simulink model "SAC_RL_env (no DEEN, orig)"  (R2025b)
settings: Solver=ode4  StartTime=0.0  StopTime=400  FixedStep=0.005  RelTol=1e-3  EnableMultiTasking=on
values from neighbouring files (symbols this model uses):
  dyn_obs = struct('p0', cell(1, num_dyn_obs), 'v', cell(1, num_dyn_obs), 'radius', cell(1, num_dyn_obs))    [genera_ostacoli_dinamici.m]    (also in visualizza_raggi_completo.m = scenario.dynamic_obstacles)
  initialGainsMultiplier = 15    [init_rl.m]    (also in report_agent.m; test.m; test_agent.m; train.m)
  is_validation = env.isValidation    [CustomSimulinkEnv.m]    (also in get_RL_env.m = evalin('base', 'is_validation'))
  logging = true    [train.m]    (also in train_agent.m; train_agent_precedente.m)
  max_angular_vel = double(pi)    [get_RL_env.m]
  max_deviazione_pos = 100    [get_RL_env.m]
  max_deviazione_vel = 20    [get_RL_env.m]
  max_distanza_goal = double(norm(initial_pos - scenario.map.q_goal))    [get_RL_env.m]
  max_vel = 30    [get_RL_env.m]
  num_rays = size(lidar_scan, 2)    [visualizza_raggi.m]
  tolleranza_goal = 2    [get_RL_env.m]
  Ts = 0.1    [init_rl.m]    (also in report_agent.m; test.m; test_agent.m; train.m)
undefined symbols (not defined in the file or in its folder): angControlTuning, angRateControlTuning, bounds, Controller, decyear, DiscIntNeverNeededParam, DroneMass, Dz, Gravity, initialConditions, Iz, leapyear, logPath_num, logPathValid_num, Nz, pos_goal, posControlTuning, Pz, startFlightTime, tunePositionController, UAVSampleTime, Vehicle, velControlTuning
libraries: slpidlib x14, slctrl_autotuning x8, sharedutil x4, matrix_library x4, aerolibconvert2 x3, aerolibatmos2 x2, aerolibgravity2 x2, shared6dof x2, aerolibasang x2, sensorinslib x2, deeplib x1, rllib x1
(part 1 of 5)
settings Model: DataDictionary=uavPackageDeliveryDataDict.sldd  ModifiedByFormat=The MathWorks, Inc.  SimulationMode=accelerator  PacingRate=0.110000  Creator=The MathWorks, Inc.  LastModifiedBy=The MathWorks, Inc.
settings SolverCC: AlgebraicLoopSolver=TrustRegion  AutoInsertRateTranBlk=on  MaxZcPerStep=1.0
settings DataIOCC: SaveOutput=off
settings OptimizationCC: LifeSpan=inf
settings DebuggingCC: ParameterPrecisionLossMsg=none  UnconnectedInputMsg=warning  UnconnectedOutputMsg=warning  UnconnectedLineMsg=warning  AllowSymbolicDim=off  SubsystemReferenceDiagnosticForUnitTest=warning  SFUnexpectedBacktrackingDiag=warning  SFNoUnconditionalDefaultTransitionDiag=warning  SFExecutionAtInitializationDiag=none  ArithmeticOperatorsInVariantConditions=warning
settings ModelReferenceCC: EnableRefExpFcnMdlSchedulingChecks=on  PropagateSignalLabelsOutOfModel=off
settings SFSimCC: SimUseLocalCustomCode=off  CustomCodeUndefinedFunction=UseInterfaceOnly
settings RTWCC: RTWUseLocalCustomCode=off  GPUComputeCapability=3.5  DLArmComputeVersion=19.05
settings CodeAppCC: StateflowObjectComments=on
settings GRTTargetCC: TargetLangStandard=C89/C90 (ANSI)
settings ConfigComp: CovMetricSettings=dw  CovSaveCumulativeToWorkspaceVar=on  CovSaveSingleToWorkspaceVar=on  CovExternalEMLEnable=off

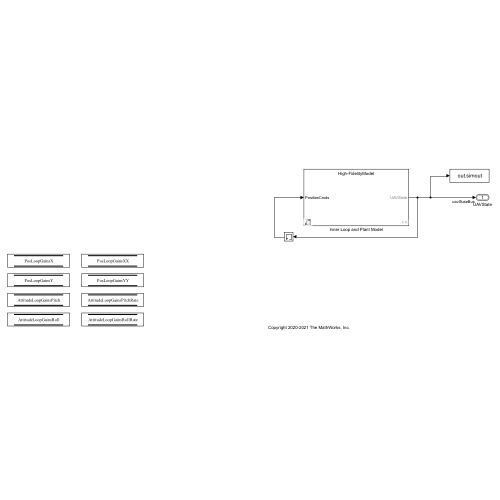
[thumbnail: Simulink's stored preview of the top-level diagram]
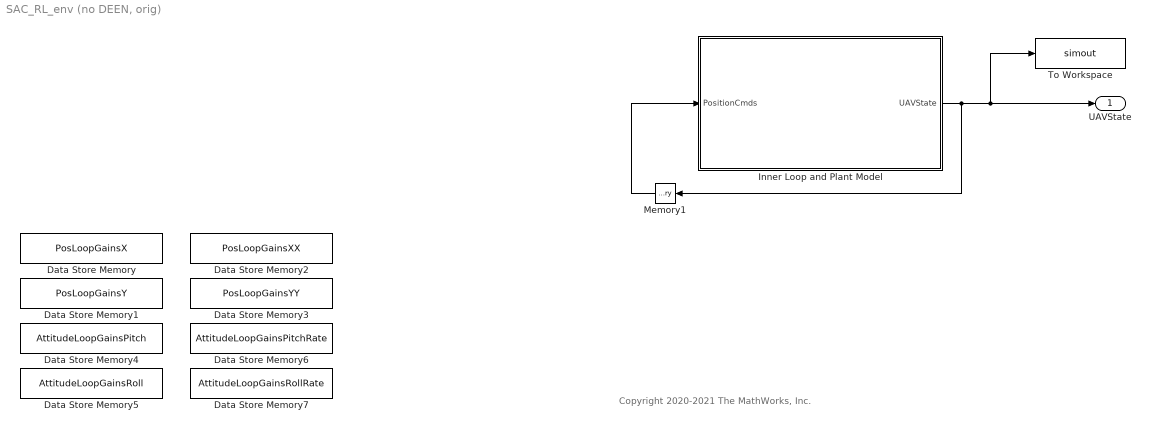
== system SAC_RL_env (no DEEN, orig) ==
  note: Copyright 2020-2021 The MathWorks, Inc.
  Data Store Memory : DataStoreMemory  DataStoreName=PosLoopGainsX  ReadBeforeWriteMsg=warning  WriteAfterWriteMsg=warning  WriteAfterReadMsg=warning  InitialValue=0.25*initialGainsMultiplier  ShowAdditionalParam=off
  Data Store Memory1 : DataStoreMemory  DataStoreName=PosLoopGainsY  ReadBeforeWriteMsg=warning  WriteAfterWriteMsg=warning  WriteAfterReadMsg=warning  InitialValue=0.25*initialGainsMultiplier  ShowAdditionalParam=off
  Data Store Memory2 : DataStoreMemory  DataStoreName=PosLoopGainsXX  ReadBeforeWriteMsg=warning  WriteAfterWriteMsg=warning  WriteAfterReadMsg=warning  InitialValue=[0.15 0.075].*initialGainsMultiplier  ShowAdditionalParam=off
  Data Store Memory3 : DataStoreMemory  DataStoreName=PosLoopGainsYY  ReadBeforeWriteMsg=warning  WriteAfterWriteMsg=warning  WriteAfterReadMsg=warning  InitialValue=[0.15 0.075].*initialGainsMultiplier  ShowAdditionalParam=off
  Data Store Memory4 : DataStoreMemory  DataStoreName=AttitudeLoopGainsPitch  ReadBeforeWriteMsg=warning  WriteAfterWriteMsg=warning  WriteAfterReadMsg=warning  InitialValue=5*initialGainsMultiplier  ShowAdditionalParam=off
  Data Store Memory5 : DataStoreMemory  DataStoreName=AttitudeLoopGainsRoll  ReadBeforeWriteMsg=warning  WriteAfterWriteMsg=warning  WriteAfterReadMsg=warning  InitialValue=5*initialGainsMultiplier  ShowAdditionalParam=off
  Data Store Memory6 : DataStoreMemory  DataStoreName=AttitudeLoopGainsPitchRate  ReadBeforeWriteMsg=warning  WriteAfterWriteMsg=warning  WriteAfterReadMsg=warning  InitialValue=[0.0025 2*0.0025 0.0025/25 70].*initialGainsMultiplier  ShowAdditionalParam=off
  Data Store Memory7 : DataStoreMemory  DataStoreName=AttitudeLoopGainsRollRate  ReadBeforeWriteMsg=warning  WriteAfterWriteMsg=warning  WriteAfterReadMsg=warning  InitialValue=[0.002 0.003 0.003/50 70].*initialGainsMultiplier  ShowAdditionalParam=off
  Inner Loop and Plant Model : Subsystem  Variant=on  PropagateVariantConditions=on
  Memory1 : Memory  InheritSampleTime=on
  To Workspace : ToWorkspace  VariableName=simout  SaveFormat=Timeseries  SampleTime=-1
  UAVState : Outport  OutDataTypeStr=Bus: uavStateBus  BusOutputAsStruct=on
  wires:
  Inner Loop and Plant Model/1(UAVState) -> Memory1/1, To Workspace/1, UAVState/1
  Memory1/1 -> Inner Loop and Plant Model/1(PositionCmds)

== system SAC_RL_env (no DEEN, orig)/Inner Loop and Plant Model ==
  PositionCmds : Inport
  High-FidelityModel : Subsystem  VariantControl=plantModelFi==1
  High-FidelityModel with Autotuning : Subsystem  VariantControl=plantModelFi==2
  Low-FidelityModel : Subsystem  VariantControl=plantModelFi ==0
  UAVState : Outport

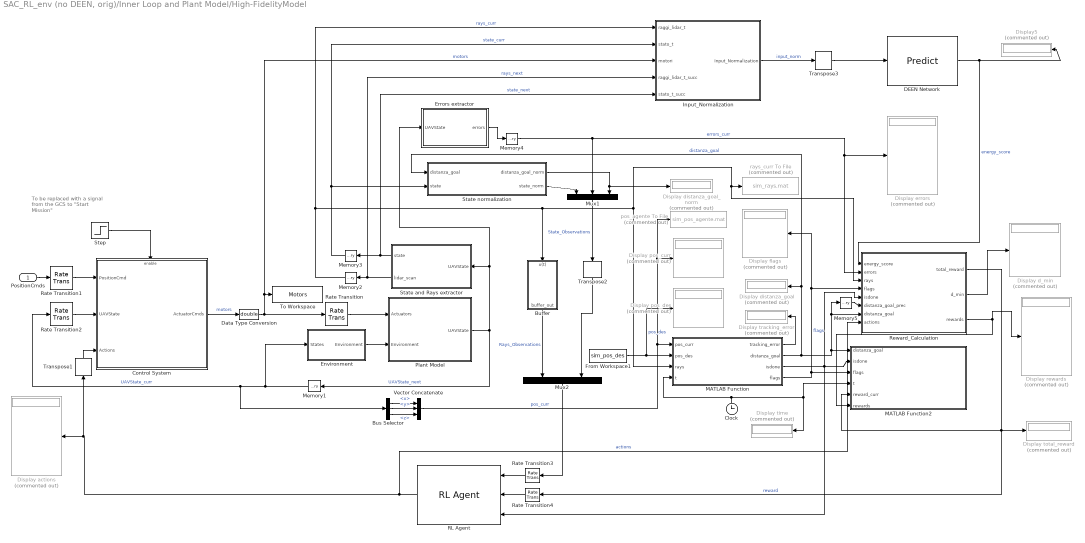
== system SAC_RL_env (no DEEN, orig)/Inner Loop and Plant Model/High-FidelityModel ==
  note: To be replaced with a signal from the GCS to "Start Mission"
  PositionCmds : Inport
  Buffer : Subsystem
  Bus Selector : BusSelector  OutputSignals=pos_vel.x,pos_vel.y,pos_vel.z
  Clock : Clock
  Control System : Subsystem  TreatAsAtomicUnit=on  SystemSampleTime=UAVSampleTime
  DEEN Network : deeplib/Predict  Network=Network from MAT-file  NetworkFunction=squeezenet  NetworkFilePath=deen_network.mat  MiniBatchSize=128  InputDataFormats={'input_transition', 'CB';}  Predictions=on  Activations={}  ForceInterpretedSim=off  EnableDLNetwork=on  LastKnownNetworkFilePath='deen_network.mat'  LastKnownNetworkTimeStamp=740118.69643518514931201934814453125
  Data Type Conversion : DataTypeConversion  OutDataTypeStr=double  SaturateOnIntegerOverflow=off  RndMeth=Floor
  Display actions : Display  Commented=on
  Display d_min : Display  Commented=on
  Display distanza_goal : Display  Commented=on
  Display distanza_goal_norm : Display  Commented=on
  Display errors : Display  Commented=on
  Display flags : Display  Commented=on
  Display pos_curr : Display  Commented=on
  Display pos_des : Display  Commented=on
  Display rewards : Display  Commented=on
  Display time : Display  Commented=on
  Display total_reward : Display  Commented=on
  Display tracking_error : Display  Commented=on
  Display5 : Display  Commented=on
  Environment : Subsystem  TreatAsAtomicUnit=on  VariantControl=VSS_ENVIRONMENT_VARIABLE
  Errors extractor : Subsystem
  From Workspace1 : FromWorkspace  VariableName=sim_pos_des
  Input_Normalization : MATLAB Function  TreatAsAtomicUnit=on
  MATLAB Function : MATLAB Function  TreatAsAtomicUnit=on
  MATLAB Function2 : MATLAB Function  TreatAsAtomicUnit=on  SystemSampleTime=Ts
  Memory{1,3..5} (4 alike) : Memory  InheritSampleTime=on  LinearizeMemory=on  LinearizeAsDelay=on
  Memory2 : Memory  InitialCondition=ones(1, num_rays)  InheritSampleTime=on  LinearizeMemory=on  LinearizeAsDelay=on
  Mux1 : Mux  Inputs=3
  Mux2 : Mux  Inputs=2
  Plant Model : Subsystem  TreatAsAtomicUnit=on
  RL Agent : rllib/RL Agent  Agent=agent  ExternalActionAsInput=off  ProvideLastAction=off  ProvideCumRwd=off  TreatAsDirectFeedthrough=on  UseStrictObservationDataTypes=off
  Rate Transition : RateTransition
  Rate Transition1 : RateTransition  OutPortSampleTime=UAVSampleTime
  Rate Transition2 : RateTransition  OutPortSampleTime=UAVSampleTime
  Rate Transition3 : RateTransition
  Rate Transition4 : RateTransition
  Reward_Calculation : MATLAB Function  TreatAsAtomicUnit=on
  State and Rays extractor : Subsystem
  State normalization : MATLAB Function  TreatAsAtomicUnit=on
  Step : Step  Time=0  SampleTime=UAVSampleTime
  To Workspace : ToWorkspace  VariableName=Motors  SaveFormat=Timeseries  SampleTime=-1
  Transpose1 : matrix_library/Transpose
  Transpose2 : matrix_library/Transpose
  Transpose3 : matrix_library/Transpose
  Vector Concatenate : Concatenate  NumInputs=3
  pos_agente To File : ToFile  Commented=on  Filename=sim_pos_agente.mat  MatrixName=sim_pos_agente  SaveFormat=Timeseries
  rays_curr To File : ToFile  Commented=on  Filename=sim_rays.mat  MatrixName=sim_rays  SaveFormat=Timeseries  SampleTime=Ts
  wires:
  PositionCmds/1 -> Rate Transition1/1
  Control System/1(ActuatorCmds) -> Data Type Conversion/1  "motors"
  Environment/1(Environment) -> Plant Model/2(Environment)
  Memory1/1 -> Bus Selector/1, Rate Transition2/1, Environment/1(States)  "UAVState_curr"
  Plant Model/1(UAVState) -> Memory1/1, State and Rays extractor/1(UAVState), Errors extractor/1(UAVState)  "UAVState_next"
  Step/1 -> Control System/Enable
  Rate Transition/1 -> Plant Model/1(Actuators)
  Rate Transition1/1 -> Control System/1(PositionCmd)
  Rate Transition2/1 -> Control System/2(UAVState)
  State and Rays extractor/2(lidar_scan) -> Input_Normalization/4(raggi_lidar_t_succ), Memory2/1  "rays_next"
  State and Rays extractor/1(state) -> Input_Normalization/5(stato_t_succ), Memory3/1  "state_next"
  Memory3/1 -> Input_Normalization/2(stato_t), State normalization/2(state)  "state_curr"
  From Workspace1/1 -> Display pos_des/1, MATLAB Function/2(pos_des)  "pos_des"
  Data Type Conversion/1 -> Input_Normalization/3(motori), To Workspace/1, Rate Transition/1  "motors"
  Bus Selector/3 -> Vector Concatenate/3  "<z>"
  Bus Selector/2 -> Vector Concatenate/2  "<y>"
  Bus Selector/1 -> Vector Concatenate/1  "<x>"
  Vector Concatenate/1 -> MATLAB Function/1(pos_curr), pos_agente To File/1, Display pos_curr/1  "pos_curr"
  RL Agent/1 -> Display actions/1, Transpose1/1, Reward_Calculation/8(actions)  "actions"
  Reward_Calculation/1(total_reward) -> Display total_reward/1, Rate Transition4/1, MATLAB Function2/5(reward_curr)  "reward"
  DEEN Network/1 -> Reward_Calculation/1(energy_score), Display5/1  "energy_score"
  Rate Transition3/1 -> RL Agent/1
  Rate Transition4/1 -> RL Agent/2
  Errors extractor/1(errors) -> Memory4/1
  Memory4/1 -> Display errors/1, Reward_Calculation/2(errors), Mux1/2  "errors_curr"
  Mux1/1 -> Transpose2/1  "State_Observations"
  Memory2/1 -> Input_Normalization/1(raggi_lidar_t), Buffer/1(x(t)), MATLAB Function/3(rays), Reward_Calculation/3(rays), rays_curr To File/1  "rays_curr"
  MATLAB Function/3(isdone) -> Reward_Calculation/5(isdone), MATLAB Function2/2(isdone), RL Agent/3
  MATLAB Function/4(flags) -> MATLAB Function2/3(flags), Display flags/1, Reward_Calculation/4(flags)  "flags"
  MATLAB Function/1(tracking_error) -> Display tracking_error/1
  Transpose1/1 -> Control System/3(Actions)
  Clock/1 -> MATLAB Function/4(t), Display time/1, MATLAB Function2/4(t)
  Buffer/1(buffer_out) -> Mux2/1  "Rays_Observations"
  Mux2/1 -> Rate Transition3/1
  State normalization/2(state_norm) -> Mux1/1
  Transpose2/1 -> Mux2/2
  Reward_Calculation/2(d_min) -> Display d_min/1
  Memory5/1 -> Reward_Calculation/6(distanza_goal_prec)
  Reward_Calculation/3(rewards) -> Display rewards/1, MATLAB Function2/6(rewards)
  Input_Normalization/1(Input_Normalization) -> Transpose3/1  "input_norm"
  MATLAB Function/2(distanza_goal) -> Display distanza_goal/1, State normalization/1(distanza_goal), Memory5/1, Reward_Calculation/7(distanza_goal), MATLAB Function2/1(distanza_goal)  "distanza_goal"
  State normalization/1(distanza_goal_norm) -> Display distanza_goal_norm/1, Mux1/3
  Transpose3/1 -> DEEN Network/1

== system SAC_RL_env (no DEEN, orig)/Inner Loop and Plant Model/High-FidelityModel with Autotuning ==
  note: To be replaced with a signal from the GCS to "Start Mission"
  PositionCmds : Inport
  Control System : Subsystem  TreatAsAtomicUnit=on  SystemSampleTime=UAVSampleTime
  Environment : Subsystem  TreatAsAtomicUnit=on  VariantControl=VSS_ENVIRONMENT_VARIABLE
  Memory1 : Memory  InheritSampleTime=on  LinearizeMemory=on  LinearizeAsDelay=on
  Plant Model : Subsystem  TreatAsAtomicUnit=on
  Rate Transition : RateTransition
  Rate Transition1 : RateTransition  OutPortSampleTime=UAVSampleTime
  Rate Transition2 : RateTransition  OutPortSampleTime=UAVSampleTime
  Step : Step  Time=startFlightTime  SampleTime=UAVSampleTime
  UAVState : Outport  OutDataTypeStr=Bus: uavStateBus
  wires:
  PositionCmds/1 -> Rate Transition1/1
  Control System/1(ActuatorCmds) -> Rate Transition/1  "motors"
  Environment/1(Environment) -> Plant Model/2(Environment)
  Memory1/1 -> Environment/1(States), Rate Transition2/1
  Plant Model/1(UAVState) -> UAVState/1, Memory1/1
  Step/1 -> Control System/Enable
  Rate Transition/1 -> Plant Model/1(Actuators)
  Rate Transition1/1 -> Control System/1(PositionCmd)
  Rate Transition2/1 -> Control System/2(UAVState)

== system SAC_RL_env (no DEEN, orig)/Inner Loop and Plant Model/Low-FidelityModel ==
  PositionCmds : Inport
  Assemble UAV State Bus : Subsystem
  Bus Creator1 : BusCreator  Inputs=1  OutDataTypeStr=Bus: uavGuidanceEnvironmentBus  NonVirtualBus=on
  Constant : Constant  Value=Gravity  OutDataTypeStr=single
      settings: AttributesFormatString=%<Value>
  Position and Acceleration Control : Subsystem
  Quadrotor Plant : uavalgslib/Guidance Model  ModelType=MultirotorGuidance  NumInstances=1  SpecifiedDataType=single  SimulateUsing=Code generation  InitialWorldPositionMultirotor=[-186; -105; 0]  InitialWorldVelocityMultirotor=[0; 0; 0]  InitialEulerZYXMultirotor=[0; 0; 0]  InitialBodyAngularRateRPYMultirotor=[0; 0; 0]  InitialThrustMultirotor=0  InitialNorthFixedWing=0  InitialEastFixedWing=0  InitialHeightFixedWing=0  InitialAirSpeedFixedWing=0  InitialHeadingAngleFixedWing=0  InitialFlightPathAngleFixedWing=0  InitialRollAngleFixedWing=0  InitialRollAngleRateFixedWing=0  PDRollMultirotor=[3402.97,116.67]  PDPitchMultirotor=[3402.97, 116.67]  PYawRateMultirotor=1950  PThrustMultirotor=39  MassMultirotor=0.1  PHeightFixedWing=3.9  PHeadingAngleFixedWing=3.9  PFlightPathAngleFixedWing=39  PDRollFixedWing=[3402.97, 116.67]  PAirSpeedFixedWing=1  FlightPathAngleLimitsFixedWing=[-pi/2, pi/2]  StateBusName='uavGuidanceStateBus'  ControlBusName='uavGuidanceControlBus'  EnvironmentBusName='uavGuidanceEnvironmentBus'  DataType=single
  Rate Transition1 : RateTransition  OutPortSampleTime=UAVSampleTime
  Rate Transition2 : RateTransition  OutPortSampleTime=UAVSampleTime
  UAVState : Outport  OutDataTypeStr=Bus: uavStateBus
  wires:
  Constant/1 -> Bus Creator1/1  "Gravity"
  Bus Creator1/1 -> Quadrotor Plant/2
  Position and Acceleration Control/1(Control Signal) -> Rate Transition2/1
  Quadrotor Plant/1 -> Rate Transition1/1
  Rate Transition2/1 -> Quadrotor Plant/1
  PositionCmds/1 -> Position and Acceleration Control/2(PositionCmd)
  Rate Transition1/1 -> Position and Acceleration Control/1(QuadRotorState), Assemble UAV State Bus/1(State)
  Assemble UAV State Bus/1(UAVState) -> UAVState/1

== system SAC_RL_env (no DEEN, orig)/Inner Loop and Plant Model/High-FidelityModel/Buffer ==
  x(t) : Inport
  Memory5 : Memory  InitialCondition=ones(1, num_rays)  InheritSampleTime=on  LinearizeMemory=on  LinearizeAsDelay=on
  Memory6 : Memory  InitialCondition=ones(1, num_rays)  InheritSampleTime=on  LinearizeMemory=on  LinearizeAsDelay=on
  Vector Concatenate1 : Concatenate  NumInputs=3
  buffer_out : Outport
  wires:
  Memory6/1 -> Vector Concatenate1/3  "x(t-2)"
  Memory5/1 -> Memory6/1, Vector Concatenate1/2  "x(t-1)"
  x(t)/1 -> Memory5/1, Vector Concatenate1/1
  Vector Concatenate1/1 -> buffer_out/1

== system SAC_RL_env (no DEEN, orig)/Inner Loop and Plant Model/High-FidelityModel/Control System ==
  note: Derived from the work by Sertac
      | Karaman and Fabian Riether
  PositionCmd : Inport
  UAVState : Inport  Port=2  BusOutputAsStruct=on
  Actions : Inport  Port=3
  Enable : EnablePort  StatesWhenEnabling=reset
  Controller : Subsystem
  ActuatorCmds : Outport  VectorParamsAs1DForOutWhenUnconnected=off
  wires:
  Controller/1(motors_refout) -> ActuatorCmds/1
  UAVState/1 -> Controller/2(UAVState)
  PositionCmd/1 -> Controller/1(PositionCmd)
  Actions/1 -> Controller/3(actions)

== system SAC_RL_env (no DEEN, orig)/Inner Loop and Plant Model/High-FidelityModel/Environment ==
  States : Inport
  Bus Creator : BusCreator  Inputs=3  OutDataTypeStr=Bus: EnvironmentBus  NonVirtualBus=on
  Bus Creator1 : BusCreator  Inputs=4  OutDataTypeStr=Bus: AtmosphereBus  NonVirtualBus=on
  Bus Selector : BusSelector  OutputSignals=gps.lat,gps.lon,gps.alt
  COESA Atmosphere Model : aerolibatmos2/COESA Atmosphere Model  units=Metric (MKS)  spec=1976 COESA-extended U.S. Standard Atmosphere  model=Profile  profile_var=High temperature  profile_percent=1%  profile_alt=5 km (16404 ft)  envelope_var=High temperature  envelope_percent=1%  action=None
  Clock : Clock
  Gain : Gain  Gain=1/1e7  OutDataTypeStr=double
  Gain1 : Gain  Gain=1/1e7  OutDataTypeStr=double
  Gain2 : Gain  Gain=1/-1e3  OutDataTypeStr=double
  Initial date : Constant  Value=decyear(initialConditions.date)
  Mux : Mux  Inputs=3
  Sum : Sum  Inputs=|++
  "WGS84 Gravity Model  " : GravityWGS84  action=None
  World Magnetic Model 2015 : aerolibgravity2/World Magnetic Model  model=WMM2015 V2 (2015-2020)  customFile='WMM2020.COF'  units=Metric (MKS)  time_in=on  month=January  day=1  year=2015  action=Error  h_out=off  dec_out=off  inc_out=off  ti_out=off
  kclock : Gain  Gain=1/(60*60*24*(365 + leapyear(initialConditions.date(1))))
  Environment : Outport  VectorParamsAs1DForOutWhenUnconnected=off
  wires:
  States/1 -> Bus Selector/1  "StatesLog"
  Bus Creator/1 -> Environment/1
  COESA Atmosphere Model/1 -> Bus Creator1/1  "air_temp"
  COESA Atmosphere Model/2 -> Bus Creator1/2  "speed_sound"
  COESA Atmosphere Model/3 -> Bus Creator1/3  "pressure"
  COESA Atmosphere Model/4 -> Bus Creator1/4  "air_density"
  Bus Creator1/1 -> Bus Creator/2  "AtmosphereBus"
  World Magnetic Model 2015/1 -> Bus Creator/3  "MagneticField_ned"
  "WGS84 Gravity Model  "/1 -> Bus Creator/1  "Gravity_ned"
  Clock/1 -> kclock/1
  Initial date/1 -> Sum/1
  Sum/1 -> World Magnetic Model 2015/4
  kclock/1 -> Sum/2
  Mux/1 -> "WGS84 Gravity Model  "/1
  Gain/1 -> World Magnetic Model 2015/2, Mux/1
  Bus Selector/1 -> Gain/1  "<lat>"
  Bus Selector/2 -> Gain1/1  "<lon>"
  Gain1/1 -> World Magnetic Model 2015/3, Mux/2
  Bus Selector/3 -> Gain2/1  "<alt>"
  Gain2/1 -> COESA Atmosphere Model/1, World Magnetic Model 2015/1, Mux/3

== system SAC_RL_env (no DEEN, orig)/Inner Loop and Plant Model/High-FidelityModel/Errors extractor ==
  UAVState : Inport
  Bus Selector3 : BusSelector  OutputSignals=pos_vel.vx,pos_vel.vy,pos_vel.vz
  Bus Selector4 : BusSelector  Commented=on  OutputSignals=attitude.yaw
  Bus Selector5 : BusSelector  OutputSignals=pos_vel.x,pos_vel.y,pos_vel.z
  Errors normalization : MATLAB Function  TreatAsAtomicUnit=on
  From Workspace3 : FromWorkspace  VariableName=sim_pos_des
  From Workspace4 : FromWorkspace  VariableName=sim_vel_des
  From Workspace5 : FromWorkspace  Commented=on  VariableName=sim_yaw_des
  Subtract : Sum  Inputs=+-
  Subtract1 : Sum  Inputs=+-
  Subtract2 : Sum  Commented=on  Inputs=+-
  Vector Concatenate5 : Concatenate
  Vector Concatenate4 : Concatenate  NumInputs=3
  Vector Concatenate6 : Concatenate  NumInputs=3
  errors : Outport  OutDataTypeStr=double
  wires:
  From Workspace4/1 -> Subtract1/1  "vel_des"
  Vector Concatenate6/1 -> Subtract/2
  Bus Selector3/1 -> Vector Concatenate4/1  "<vx>"
  Bus Selector3/2 -> Vector Concatenate4/2  "<vy>"
  Vector Concatenate4/1 -> Subtract1/2
  From Workspace3/1 -> Subtract/1
  Bus Selector5/1 -> Vector Concatenate6/1  "<x>"
  From Workspace5/1 -> Subtract2/1  "yaw_des"
  Bus Selector4/1 -> Subtract2/2  "<yaw>"
  Bus Selector5/3 -> Vector Concatenate6/3  "<z>"
  UAVState/1 -> Bus Selector5/1, Bus Selector3/1, Bus Selector4/1
  Subtract1/1 -> Vector Concatenate5/2  "errore_vel"
  Subtract/1 -> Vector Concatenate5/1  "errore_pos"
  Bus Selector5/2 -> Vector Concatenate6/2  "<y>"
  Vector Concatenate5/1 -> Errors normalization/1(errors)
  Bus Selector3/3 -> Vector Concatenate4/3  "<vz>"
  Subtract2/1 -> ?  "errore_yaw"
  Errors normalization/1(errors_normalized) -> errors/1

== system SAC_RL_env (no DEEN, orig)/Inner Loop and Plant Model/High-FidelityModel/Plant Model ==
  Actuators : Inport
  Environment : Inport  Port=2
  6DOF (Quaternion) : shared6dof/6DOF (Euler Angles)  units=Metric (MKS)  mtype=Fixed  rep=Euler Angles  xme_0=init_pos  Vm_0=[0 0 0]  eul_0=[0,0,0]  pm_0=[0,0,0]  mass_0=Vehicle.Airframe.mass  mass_e=0.5  mass_f=2.0  inertia=Vehicle.Airframe.inertia  inertia_e=eye(3)  inertia_f=2*eye(3)  k_quat=Vehicle.SixDOF.quatGain  vre_flag=on  abi_flag=on  aMode=aMode  xme_statename=''  Vm_statename=''  eul_statename=''  quat_statename=''  pm_statename=''  mass_statename=''
  AC model : Subsystem
  Bus setup : Subsystem
  Direction Cosine Matrix to Quaternions : Dcm2Quat
  Terminator1 : Terminator
  Terminator2 : Terminator
  Terminator3 : Terminator
  To Workspace : ToWorkspace  VariableName=quat_sim  SaveFormat=Timeseries  SampleTime=-1
  UAVState : Outport  VectorParamsAs1DForOutWhenUnconnected=off
  wires:
  Actuators/1 -> AC model/1(Actuators)
  Environment/1 -> AC model/2(Environment)
  AC model/1(F_cg) -> 6DOF (Quaternion)/1
  AC model/2(M_cg) -> 6DOF (Quaternion)/2
  6DOF (Quaternion)/1 -> Bus setup/1(V_ned)
  6DOF (Quaternion)/2 -> Bus setup/2(X_ned)
  6DOF (Quaternion)/3 -> Bus setup/3(Euler)
  6DOF (Quaternion)/6 -> Bus setup/5(Omega_b), AC model/5(w_b)
  6DOF (Quaternion)/5 -> AC model/4(V_b)
  6DOF (Quaternion)/4 -> Bus setup/4(DCM), Direction Cosine Matrix to Quaternions/1, AC model/3(DCM_be)
  Bus setup/1(UAVState) -> UAVState/1
  6DOF (Quaternion)/9 -> Terminator1/1
  6DOF (Quaternion)/7 -> Terminator2/1
  6DOF (Quaternion)/8 -> Terminator3/1
  Direction Cosine Matrix to Quaternions/1 -> To Workspace/1

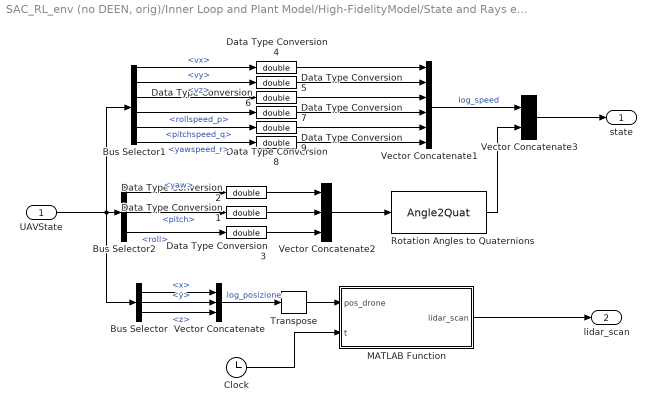
== system SAC_RL_env (no DEEN, orig)/Inner Loop and Plant Model/High-FidelityModel/State and Rays extractor ==
  UAVState : Inport
  Bus Selector : BusSelector  OutputSignals=pos_vel.x,pos_vel.y,pos_vel.z
  Bus Selector1 : BusSelector  OutputSignals=pos_vel.vx,pos_vel.vy,pos_vel.vz,attitude.rollspeed_p,attitude.pitchspeed_q,attitude.yawspeed_r
  Bus Selector2 : BusSelector  OutputSignals=attitude.yaw,attitude.pitch,attitude.roll
  Clock : Clock
  Data Type Conversion{1..9} (9 alike) : DataTypeConversion  OutDataTypeStr=double  SaturateOnIntegerOverflow=off  RndMeth=Floor
  MATLAB Function : MATLAB Function  TreatAsAtomicUnit=on
  Rotation Angles to Quaternions : Angle2Quat
      settings: AttributesFormatString=Rotation Order: %<rotationOrder>
  Transpose : matrix_library/Transpose
  Vector Concatenate : Concatenate  NumInputs=3
  Vector Concatenate1 : Concatenate  NumInputs=6
  Vector Concatenate2 : Concatenate  NumInputs=3
  Vector Concatenate3 : Concatenate
  state : Outport  OutDataTypeStr=double
  lidar_scan : Outport  Port=2  OutDataTypeStr=double
  wires:
  Vector Concatenate1/1 -> Vector Concatenate3/1  "log_speed"
  Bus Selector1/1 -> Data Type Conversion4/1  "<vx>"
  Rotation Angles to Quaternions/1 -> Vector Concatenate3/2
  Bus Selector1/4 -> Data Type Conversion7/1  "<rollspeed_p>"
  UAVState/1 -> Bus Selector2/1, Bus Selector/1, Bus Selector1/1
  Bus Selector1/2 -> Data Type Conversion5/1  "<vy>"
  Bus Selector1/5 -> Data Type Conversion8/1  "<pitchspeed_q>"
  Vector Concatenate/1 -> Transpose/1  "log_posizione"
  Bus Selector/1 -> Vector Concatenate/1  "<x>"
  Bus Selector1/3 -> Data Type Conversion6/1  "<vz>"
  Bus Selector1/6 -> Data Type Conversion9/1  "<yawspeed_r>"
  Vector Concatenate2/1 -> Rotation Angles to Quaternions/1
  Bus Selector/3 -> Vector Concatenate/3  "<z>"
  Bus Selector/2 -> Vector Concatenate/2  "<y>"
  Vector Concatenate3/1 -> state/1
  Bus Selector2/2 -> Data Type Conversion1/1  "<pitch>"
  Data Type Conversion1/1 -> Vector Concatenate2/2
  Bus Selector2/1 -> Data Type Conversion2/1  "<yaw>"
  Data Type Conversion2/1 -> Vector Concatenate2/1
  Data Type Conversion3/1 -> Vector Concatenate2/3
  Bus Selector2/3 -> Data Type Conversion3/1  "<roll>"
  Data Type Conversion4/1 -> Vector Concatenate1/1
  Data Type Conversion5/1 -> Vector Concatenate1/2
  Data Type Conversion6/1 -> Vector Concatenate1/3
  Data Type Conversion7/1 -> Vector Concatenate1/4
  Data Type Conversion8/1 -> Vector Concatenate1/5
  Data Type Conversion9/1 -> Vector Concatenate1/6
  Transpose/1 -> MATLAB Function/1(pos_drone)
  Clock/1 -> MATLAB Function/2(t)
  MATLAB Function/1(lidar_scan) -> lidar_scan/1

== system SAC_RL_env (no DEEN, orig)/Inner Loop and Plant Model/High-FidelityModel with Autotuning/Control System ==
  note: Derived from the work by Sertac
      | Karaman and Fabian Riether
  PositionCmd : Inport
  UAVState : Inport  Port=2  BusOutputAsStruct=on
  Enable : EnablePort  StatesWhenEnabling=reset
  Controller : Subsystem
  ActuatorCmds : Outport  VectorParamsAs1DForOutWhenUnconnected=off
  wires:
  Controller/1(motors_refout) -> ActuatorCmds/1
  UAVState/1 -> Controller/2(UAVState)
  PositionCmd/1 -> Controller/1(PositionCmd)

== system SAC_RL_env (no DEEN, orig)/Inner Loop and Plant Model/High-FidelityModel with Autotuning/Environment ==
  States : Inport
  Bus Creator : BusCreator  Inputs=3  OutDataTypeStr=Bus: EnvironmentBus  NonVirtualBus=on
  Bus Creator1 : BusCreator  Inputs=4  OutDataTypeStr=Bus: AtmosphereBus  NonVirtualBus=on
  Bus Selector : BusSelector  OutputSignals=gps.lat,gps.lon,gps.alt
  COESA Atmosphere Model : aerolibatmos2/COESA Atmosphere Model  units=Metric (MKS)  spec=1976 COESA-extended U.S. Standard Atmosphere  model=Profile  profile_var=High temperature  profile_percent=1%  profile_alt=5 km (16404 ft)  envelope_var=High temperature  envelope_percent=1%  action=None
  Clock : Clock
  Gain : Gain  Gain=1/1e7  OutDataTypeStr=double
  Gain1 : Gain  Gain=1/1e7  OutDataTypeStr=double
  Gain2 : Gain  Gain=1/-1e3  OutDataTypeStr=double
  Initial date : Constant  Value=decyear(initialConditions.date)
  Mux : Mux  Inputs=3
  Sum : Sum  Inputs=|++
  "WGS84 Gravity Model  " : GravityWGS84  action=None
  World Magnetic Model 2015 : aerolibgravity2/World Magnetic Model  model=WMM2015 V2 (2015-2020)  customFile='WMM2020.COF'  units=Metric (MKS)  time_in=on  month=January  day=1  year=2015  action=Error  h_out=off  dec_out=off  inc_out=off  ti_out=off
  kclock : Gain  Gain=1/(60*60*24*(365 + leapyear(initialConditions.date(1))))
  Environment : Outport  VectorParamsAs1DForOutWhenUnconnected=off
  wires:
  States/1 -> Bus Selector/1  "StatesLog"
  Bus Creator/1 -> Environment/1
  COESA Atmosphere Model/1 -> Bus Creator1/1  "air_temp"
  COESA Atmosphere Model/2 -> Bus Creator1/2  "speed_sound"
  COESA Atmosphere Model/3 -> Bus Creator1/3  "pressure"
  COESA Atmosphere Model/4 -> Bus Creator1/4  "air_density"
  Bus Creator1/1 -> Bus Creator/2  "AtmosphereBus"
  World Magnetic Model 2015/1 -> Bus Creator/3  "MagneticField_ned"
  "WGS84 Gravity Model  "/1 -> Bus Creator/1  "Gravity_ned"
  Clock/1 -> kclock/1
  Initial date/1 -> Sum/1
  Sum/1 -> World Magnetic Model 2015/4
  kclock/1 -> Sum/2
  Mux/1 -> "WGS84 Gravity Model  "/1
  Gain/1 -> World Magnetic Model 2015/2, Mux/1
  Bus Selector/1 -> Gain/1  "<lat>"
  Bus Selector/2 -> Gain1/1  "<lon>"
  Gain1/1 -> World Magnetic Model 2015/3, Mux/2
  Bus Selector/3 -> Gain2/1  "<alt>"
  Gain2/1 -> COESA Atmosphere Model/1, World Magnetic Model 2015/1, Mux/3

== system SAC_RL_env (no DEEN, orig)/Inner Loop and Plant Model/High-FidelityModel with Autotuning/Plant Model ==
  Actuators : Inport
  Environment : Inport  Port=2
  6DOF (Quaternion) : shared6dof/6DOF (Euler Angles)  units=Metric (MKS)  mtype=Fixed  rep=Euler Angles  xme_0=initialConditions.posNED + [0 0 -1]  Vm_0=[0 0 0]  eul_0=[0,0,0]  pm_0=[0,0,0]  mass_0=Vehicle.Airframe.mass  mass_e=0.5  mass_f=2.0  inertia=Vehicle.Airframe.inertia  inertia_e=eye(3)  inertia_f=2*eye(3)  k_quat=Vehicle.SixDOF.quatGain  vre_flag=on  abi_flag=on  aMode=aMode  xme_statename=''  Vm_statename=''  eul_statename=''  quat_statename=''  pm_statename=''  mass_statename=''
  AC model : Subsystem
  Bus setup : Subsystem
  Terminator1 : Terminator
  Terminator2 : Terminator
  Terminator3 : Terminator
  UAVState : Outport  VectorParamsAs1DForOutWhenUnconnected=off
  wires:
  Actuators/1 -> AC model/1(Actuators)
  Environment/1 -> AC model/2(Environment)
  AC model/1(F_cg) -> 6DOF (Quaternion)/1
  AC model/2(M_cg) -> 6DOF (Quaternion)/2
  6DOF (Quaternion)/1 -> Bus setup/1(V_ned)
  6DOF (Quaternion)/2 -> Bus setup/2(X_ned)
  6DOF (Quaternion)/3 -> Bus setup/3(Euler)
  6DOF (Quaternion)/6 -> Bus setup/5(Omega_b), AC model/5(w_b)
  6DOF (Quaternion)/5 -> AC model/4(V_b)
  6DOF (Quaternion)/4 -> Bus setup/4(DCM), AC model/3(DCM_be)
  Bus setup/1(UAVState) -> UAVState/1
  6DOF (Quaternion)/9 -> Terminator1/1
  6DOF (Quaternion)/7 -> Terminator2/1
  6DOF (Quaternion)/8 -> Terminator3/1

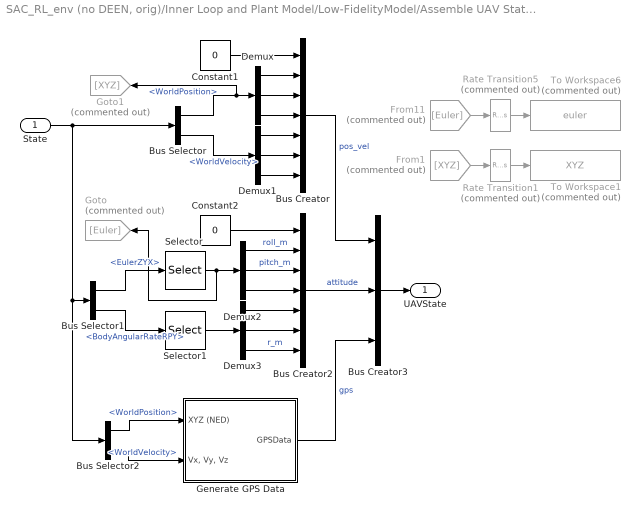
== system SAC_RL_env (no DEEN, orig)/Inner Loop and Plant Model/Low-FidelityModel/Assemble UAV State Bus ==
  State : Inport
  Bus Creator : BusCreator  Inputs=7  OutDataTypeStr=Bus: local_position_ned
      settings: InheritFromInputs=off
  Bus Creator2 : BusCreator  Inputs=7  OutDataTypeStr=Bus: attitudeBus
      settings: InheritFromInputs=off
  Bus Creator3 : BusCreator  Inputs=3  OutDataTypeStr=Bus: uavStateBus
      settings: InheritFromInputs=off
  Bus Selector : BusSelector  OutputSignals=WorldPosition,WorldVelocity
  Bus Selector1 : BusSelector  OutputSignals=EulerZYX,BodyAngularRateRPY
  Bus Selector2 : BusSelector  OutputSignals=WorldPosition,WorldVelocity
  Constant1 : Constant  Value=0  OutDataTypeStr=uint32
  Constant2 : Constant  Value=0  OutDataTypeStr=uint32
  Demux{,1..3} (4 alike) : Demux  Outputs=3
  From1 : From  Commented=on  GotoTag=XYZ
  From11 : From  Commented=on  GotoTag=Euler
  Generate GPS Data : Subsystem
  Goto : Goto  Commented=on  GotoTag=Euler
  Goto1 : Goto  Commented=on  GotoTag=XYZ
  Rate Transition1 : RateTransition  Commented=on  OutPortSampleTime=UAVSampleTime
  Rate Transition5 : RateTransition  Commented=on  OutPortSampleTime=UAVSampleTime
  Selector : Selector  InputPortWidth=3  IndexOptions=Index vector (dialog)  Indices=[3 2 1]  OutputSizes=1
  Selector1 : Selector  InputPortWidth=3  IndexOptions=Index vector (dialog)  Indices=[3 2 1]  OutputSizes=1
  To Workspace1 : ToWorkspace  Commented=on  VariableName=XYZ  SaveFormat=Timeseries  SampleTime=-1
  To Workspace6 : ToWorkspace  Commented=on  VariableName=euler  SaveFormat=Timeseries  SampleTime=-1
  UAVState : Outport  OutDataTypeStr=Bus: uavStateBus
  wires:
  Bus Creator2/1 -> Bus Creator3/2  "attitude"
  Bus Creator3/1 -> UAVState/1
  Demux3/1 -> Bus Creator2/5
  Demux1/2 -> Bus Creator/6
  Bus Creator/1 -> Bus Creator3/1  "pos_vel"
  Demux1/3 -> Bus Creator/7
  Bus Selector2/2 -> Generate GPS Data/2("Vx, Vy, Vz")  "<WorldVelocity>"
  Demux/1 -> Bus Creator/2
  State/1 -> Bus Selector/1, Bus Selector2/1, Bus Selector1/1
  Constant2/1 -> Bus Creator2/1
  Bus Selector/1 -> Goto1/1, Demux/1  "<WorldPosition>"
  Selector1/1 -> Demux3/1
  Demux1/1 -> Bus Creator/5
  Bus Selector1/1 -> Selector/1  "<EulerZYX>"
  Demux/2 -> Bus Creator/3
  Demux2/1 -> Bus Creator2/2  "roll_m"
  Demux2/3 -> Bus Creator2/4
  Demux3/2 -> Bus Creator2/6
  Demux2/2 -> Bus Creator2/3  "pitch_m"
  Bus Selector1/2 -> Selector1/1  "<BodyAngularRateRPY>"
  Demux3/3 -> Bus Creator2/7  "r_m"
  Demux/3 -> Bus Creator/4
  Bus Selector/2 -> Demux1/1  "<WorldVelocity>"
  Constant1/1 -> Bus Creator/1
  Bus Selector2/1 -> Generate GPS Data/1(XYZ (NED))  "<WorldPosition>"
  Generate GPS Data/1(GPSData) -> Bus Creator3/3  "gps"
  Rate Transition5/1 -> To Workspace6/1
  From11/1 -> Rate Transition5/1
  Selector/1 -> Goto/1, Demux2/1
  From1/1 -> Rate Transition1/1
  Rate Transition1/1 -> To Workspace1/1

== system SAC_RL_env (no DEEN, orig)/Inner Loop and Plant Model/Low-FidelityModel/Position and Acceleration Control ==
  note: To be replaced with a signal from the GCS to "Start Mission"
  QuadRotorState : Inport
  PositionCmd : Inport  Port=2
  Attitude Control : Subsystem
  Position Control : Subsystem
  Step : Step  Time=startFlightTime  SampleTime=UAVSampleTime
  Velocity Control : Subsystem
  Control Signal : Outport
  wires:
  PositionCmd/1 -> Position Control/1(PositionCmd), Attitude Control/3(PositionCmd)
  Velocity Control/1(Accel Cmd) -> Attitude Control/1(Accel Cmd)
  Attitude Control/1(Control Signal) -> Control Signal/1
  QuadRotorState/1 -> Velocity Control/2(QuadRotorState), Attitude Control/2(QuadRotorState), Position Control/2(QuadRotorState)
  Position Control/1(Velocity Cmd) -> Velocity Control/1(Velocity Cmd)
  Step/1 -> Velocity Control/Enable, Position Control/Enable

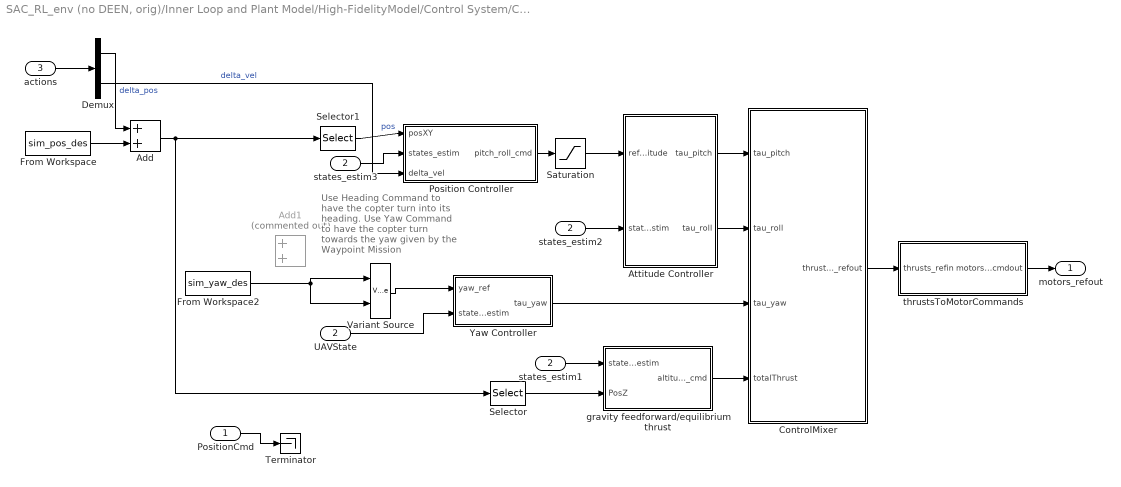
== system SAC_RL_env (no DEEN, orig)/Inner Loop and Plant Model/High-FidelityModel/Control System/Controller ==
  note: Use Heading Command to have
      | the copter turn into its heading.
      | Use Yaw Command to have the
      | copter turn towards the yaw given
      | by the Waypoint Mission
  PositionCmd : Inport
  UAVState : Inport  Port=2
  actions : Inport  Port=3
  Add : Sum
  Add1 : Sum  Commented=on
  Attitude Controller : Subsystem
  ControlMixer : Subsystem
  Demux : Demux  Outputs=[3, 3]
  From Workspace : FromWorkspace  VariableName=sim_pos_des
  From Workspace2 : FromWorkspace  VariableName=sim_yaw_des
  Position Controller : Subsystem
  Saturation : Saturate
  Selector : Selector  InputPortWidth=3  IndexOptions=Index vector (dialog)  Indices=3  OutputSizes=1
  Selector1 : Selector  InputPortWidth=3  IndexOptions=Index vector (dialog)  Indices=[1 2]  OutputSizes=1
  Terminator : Terminator
  Variant Source : VariantSource  VariantControls={useHeading ==1, useHeading~=1}
  Yaw Controller : Subsystem
  gravity feedforward/equilibrium thrust : Subsystem
  states_estim1 : InportShadow  Port=2
  states_estim2 : InportShadow  Port=2
  states_estim3 : InportShadow  Port=2
  thrustsToMotorCommands : Subsystem
  motors_refout : Outport  VectorParamsAs1DForOutWhenUnconnected=off
  wires:
  Yaw Controller/1(tau_yaw) -> ControlMixer/3(tau_yaw)
  thrustsToMotorCommands/1(motors_cmdout) -> motors_refout/1
  states_estim3/1 -> Position Controller/2(states_estim)
  ControlMixer/1(thrusts_refout) -> thrustsToMotorCommands/1(thrusts_refin)
  gravity feedforward/equilibrium thrust/1(altitude_cmd) -> ControlMixer/4(totalThrust)
  Selector1/1 -> Position Controller/1(posXY)  "pos"
  states_estim1/1 -> gravity feedforward/equilibrium thrust/1(states_estim)
  UAVState/1 -> Yaw Controller/2(states_estim)
  states_estim2/1 -> Attitude Controller/2(states_estim)
  Selector/1 -> gravity feedforward/equilibrium thrust/2(PosZ)
  Attitude Controller/1(tau_pitch) -> ControlMixer/1(tau_pitch)
  Attitude Controller/2(tau_roll) -> ControlMixer/2(tau_roll)
  Position Controller/1(pitch_roll_cmd) -> Saturation/1
  Variant Source/1 -> Yaw Controller/1(yaw_ref)
  PositionCmd/1 -> Terminator/1
  Saturation/1 -> Attitude Controller/1(refAttitude)
  From Workspace/1 -> Add/2
  Add/1 -> Selector/1, Selector1/1
  Demux/2 -> Position Controller/3(delta_vel)  "delta_vel"
  Demux/1 -> Add/1  "delta_pos"
  ? -> Add1/1  "delta_yaw"
  From Workspace2/1 -> Variant Source/1, Variant Source/2
  actions/1 -> Demux/1

== system SAC_RL_env (no DEEN, orig)/Inner Loop and Plant Model/High-FidelityModel/Plant Model/AC model ==
  Actuators : Inport
  Environment : Inport  Port=2
  DCM_be : Inport  Port=3
  V_b : Inport  Port=4  Unit=m/s
  w_b : Inport  Port=5  Unit=rad/s
  Applied Force Calculation : Subsystem
  Bus Selector : BusSelector  OutputSignals=Gravity_ned,AtmosphereBus.air_density
  Drag Calculation : Subsystem
  Gravity Force Calculation : Subsystem
  Motor Forces and Torques : Subsystem
  F_cg : Outport  Unit=N  VectorParamsAs1DForOutWhenUnconnected=off
  M_cg : Outport  Port=2  Unit=N*m  VectorParamsAs1DForOutWhenUnconnected=off
  wires:
  Applied Force Calculation/1(External Forces) -> F_cg/1
  Motor Forces and Torques/2(Motor Torques) -> M_cg/1
  Motor Forces and Torques/1(Motor Forces) -> Applied Force Calculation/3(Motor Forces)
  Bus Selector/1 -> Gravity Force Calculation/2(gravity)  "<Gravity_ned>"
  Gravity Force Calculation/1(gravity force) -> Applied Force Calculation/1(gravity force)
  Environment/1 -> Bus Selector/1
  Bus Selector/2 -> Motor Forces and Torques/2(Density), Drag Calculation/1(Density)  "<air_density>"
  DCM_be/1 -> Gravity Force Calculation/1(DCMbe)
  V_b/1 -> Motor Forces and Torques/1(Vb), Drag Calculation/2(Vb)
  Drag Calculation/1(Drag) -> Applied Force Calculation/2(Aerodynamic Forces)
  Actuators/1 -> Motor Forces and Torques/4(Motor Commands)
  w_b/1 -> Motor Forces and Torques/3(pqr)

== system SAC_RL_env (no DEEN, orig)/Inner Loop and Plant Model/High-FidelityModel/Plant Model/Bus setup ==
  V_ned : Inport  Unit=m/second  PortDimensions=3
  X_ned : Inport  Port=2  Unit=m  PortDimensions=3
  Euler : Inport  Port=3  Unit=rad  PortDimensions=3
  DCM : Inport  Port=4
  Omega_b : Inport  Port=5  Unit=rad/s  PortDimensions=3
  Bus Creator : BusCreator  Inputs=7  OutDataTypeStr=Bus: local_position_ned
      settings: InheritFromInputs=off
  Bus Creator2 : BusCreator  Inputs=7  OutDataTypeStr=Bus: attitudeBus
      settings: InheritFromInputs=off
  Bus Creator3 : BusCreator  Inputs=3  OutDataTypeStr=Bus: uavStateBus
      settings: InheritFromInputs=off
  Constant1 : Constant  Value=0  OutDataTypeStr=uint32
  Constant2 : Constant  Value=0  OutDataTypeStr=uint32
  Data Type Conversion{,1..4} (5 alike) : DataTypeConversion  OutDataTypeStr=single  SaturateOnIntegerOverflow=off  RndMeth=Floor
  Demux{,1..3} (4 alike) : Demux  Outputs=3
  Generate GPS Data : Subsystem
  UAVState : Outport  OutDataTypeStr=Bus: uavStateBus
  wires:
  Demux1/3 -> Bus Creator/7
  Bus Creator3/1 -> UAVState/1
  Demux/2 -> Bus Creator/3
  Demux3/2 -> Bus Creator2/6
  Bus Creator2/1 -> Bus Creator3/2  "attitude"
  Demux1/2 -> Bus Creator/6
  Demux3/1 -> Bus Creator2/5
  Demux/1 -> Bus Creator/2
  Euler/1 -> Data Type Conversion1/1
  Demux2/3 -> Bus Creator2/4
  Demux2/1 -> Bus Creator2/2  "roll_m"
  Bus Creator/1 -> Bus Creator3/1  "pos_vel"
  Constant2/1 -> Bus Creator2/1
  Demux2/2 -> Bus Creator2/3  "pitch_m"
  Demux3/3 -> Bus Creator2/7  "r_m"
  Demux1/1 -> Bus Creator/5
  V_ned/1 -> Data Type Conversion3/1
  Omega_b/1 -> Data Type Conversion2/1
  Demux/3 -> Bus Creator/4
  Constant1/1 -> Bus Creator/1
  Generate GPS Data/1(GPSData) -> Bus Creator3/3  "gps"
  X_ned/1 -> Data Type Conversion/1
  Data Type Conversion/1 -> Generate GPS Data/1(XYZ (NEU)), Demux/1
  Data Type Conversion2/1 -> Demux3/1
  Data Type Conversion1/1 -> Demux2/1
  Data Type Conversion3/1 -> Demux1/1, Generate GPS Data/2("Vx, Vy, Vz")
  DCM/1 -> Data Type Conversion4/1
  Data Type Conversion4/1 -> Generate GPS Data/3(DCM)

== system SAC_RL_env (no DEEN, orig)/Inner Loop and Plant Model/High-FidelityModel with Autotuning/Control System/Controller ==
  note: Use Heading Command to have
      | the copter turn into its heading.
      | Use Yaw Command to have the
      | copter turn towards the yaw given
      | by the Waypoint Mission
  In Bus Element2 : Inport  PortName=PositionCmd  Element=LAP
  In Bus Element : Inport  PortName=PositionCmd  Element=LAP
  In Bus Element3 : Inport  PortName=PositionCmd  Element=YawCmd
  In Bus Element1 : Inport  PortName=PositionCmd  Element=HeadingCmd
  UAVState : Inport  Port=2
  Attitude Controller : Subsystem
  ControlMixer : Subsystem
  Position Controller : Subsystem
  Selector : Selector  InputPortWidth=3  IndexOptions=Index vector (dialog)  Indices=3  OutputSizes=1
  Selector1 : Selector  InputPortWidth=3  IndexOptions=Index vector (dialog)  Indices=[1 2]  OutputSizes=1
  Variant Source : VariantSource  VariantControls={useHeading ==1, useHeading~=1}
  Yaw Controller : Subsystem
  gravity feedforward/equilibrium thrust : Subsystem
  states_estim1 : InportShadow  Port=2
  states_estim2 : InportShadow  Port=2
  states_estim3 : InportShadow  Port=2
  thrustsToMotorCommands : Subsystem
  motors_refout : Outport  VectorParamsAs1DForOutWhenUnconnected=off
  wires:
  Yaw Controller/1(tau_yaw) -> ControlMixer/3(tau_yaw)
  thrustsToMotorCommands/1(motors_cmdout) -> motors_refout/1
  states_estim3/1 -> Position Controller/2(states_estim)
  ControlMixer/1(thrusts_refout) -> thrustsToMotorCommands/1(thrusts_refin)
  gravity feedforward/equilibrium thrust/1(altitude_cmd) -> ControlMixer/4(totalThrust)
  Selector1/1 -> Position Controller/1(posXY)  "pos"
  states_estim1/1 -> gravity feedforward/equilibrium thrust/1(states_estim)
  UAVState/1 -> Yaw Controller/2(states_estim)
  states_estim2/1 -> Attitude Controller/2(states_estim)
  In Bus Element2/1 -> Selector1/1
  In Bus Element/1 -> Selector/1
  Selector/1 -> gravity feedforward/equilibrium thrust/2(PosZ)
  Attitude Controller/1(tau_pitch) -> ControlMixer/1(tau_pitch)
  Attitude Controller/2(tau_roll) -> ControlMixer/2(tau_roll)
  In Bus Element3/1 -> Variant Source/2
  Position Controller/1(pitch_roll_cmd) -> Attitude Controller/1(refAttitude)
  Variant Source/1 -> Yaw Controller/1(yaw_ref)
  In Bus Element1/1 -> Variant Source/1

== system SAC_RL_env (no DEEN, orig)/Inner Loop and Plant Model/High-FidelityModel with Autotuning/Plant Model/AC model ==
  Actuators : Inport
  Environment : Inport  Port=2
  DCM_be : Inport  Port=3
  V_b : Inport  Port=4  Unit=m/s
  w_b : Inport  Port=5  Unit=rad/s
  Applied Force Calculation : Subsystem
  Bus Selector : BusSelector  OutputSignals=Gravity_ned,AtmosphereBus.air_density
  Drag Calculation : Subsystem
  Gravity Force Calculation : Subsystem
  Motor Forces and Torques : Subsystem
  F_cg : Outport  Unit=N  VectorParamsAs1DForOutWhenUnconnected=off
  M_cg : Outport  Port=2  Unit=N*m  VectorParamsAs1DForOutWhenUnconnected=off
  wires:
  Applied Force Calculation/1(External Forces) -> F_cg/1
  Motor Forces and Torques/2(Motor Torques) -> M_cg/1
  Motor Forces and Torques/1(Motor Forces) -> Applied Force Calculation/3(Motor Forces)
  Bus Selector/1 -> Gravity Force Calculation/2(gravity)  "<Gravity_ned>"
  Gravity Force Calculation/1(gravity force) -> Applied Force Calculation/1(gravity force)
  Environment/1 -> Bus Selector/1
  Bus Selector/2 -> Motor Forces and Torques/2(Density), Drag Calculation/1(Density)  "<air_density>"
  DCM_be/1 -> Gravity Force Calculation/1(DCMbe)
  V_b/1 -> Motor Forces and Torques/1(Vb), Drag Calculation/2(Vb)
  Drag Calculation/1(Drag) -> Applied Force Calculation/2(Aerodynamic Forces)
  Actuators/1 -> Motor Forces and Torques/4(Motor Commands)
  w_b/1 -> Motor Forces and Torques/3(pqr)

== system SAC_RL_env (no DEEN, orig)/Inner Loop and Plant Model/High-FidelityModel with Autotuning/Plant Model/Bus setup ==
  V_ned : Inport  Unit=m/second  PortDimensions=3
  X_ned : Inport  Port=2  Unit=m  PortDimensions=3
  Euler : Inport  Port=3  Unit=rad  PortDimensions=3
  DCM : Inport  Port=4
  Omega_b : Inport  Port=5  Unit=rad/s  PortDimensions=3
  Bus Creator : BusCreator  Inputs=7  OutDataTypeStr=Bus: local_position_ned
      settings: InheritFromInputs=off
  Bus Creator2 : BusCreator  Inputs=7  OutDataTypeStr=Bus: attitudeBus
      settings: InheritFromInputs=off
  Bus Creator3 : BusCreator  Inputs=3  OutDataTypeStr=Bus: uavStateBus
      settings: InheritFromInputs=off
  Constant1 : Constant  Value=0  OutDataTypeStr=uint32
  Constant2 : Constant  Value=0  OutDataTypeStr=uint32
  Data Type Conversion{,1..4} (5 alike) : DataTypeConversion  OutDataTypeStr=single  SaturateOnIntegerOverflow=off  RndMeth=Floor
  Demux{,1..3} (4 alike) : Demux  Outputs=3
  Generate GPS Data : Subsystem
  UAVState : Outport  OutDataTypeStr=Bus: uavStateBus
  wires:
  Demux1/3 -> Bus Creator/7
  Bus Creator3/1 -> UAVState/1
  Demux/2 -> Bus Creator/3
  Demux3/2 -> Bus Creator2/6
  Bus Creator2/1 -> Bus Creator3/2  "attitude"
  Demux1/2 -> Bus Creator/6
  Demux3/1 -> Bus Creator2/5
  Demux/1 -> Bus Creator/2
  Euler/1 -> Data Type Conversion1/1
  Demux2/3 -> Bus Creator2/4
  Demux2/1 -> Bus Creator2/2  "roll_m"
  Bus Creator/1 -> Bus Creator3/1  "pos_vel"
  Constant2/1 -> Bus Creator2/1
  Demux2/2 -> Bus Creator2/3  "pitch_m"
  Demux3/3 -> Bus Creator2/7  "r_m"
  Demux1/1 -> Bus Creator/5
  V_ned/1 -> Data Type Conversion3/1
  Omega_b/1 -> Data Type Conversion2/1
  Demux/3 -> Bus Creator/4
  Constant1/1 -> Bus Creator/1
  Generate GPS Data/1(GPSData) -> Bus Creator3/3  "gps"
  X_ned/1 -> Data Type Conversion/1
  Data Type Conversion/1 -> Generate GPS Data/1(XYZ (NEU)), Demux/1
  Data Type Conversion2/1 -> Demux3/1
  Data Type Conversion1/1 -> Demux2/1
  Data Type Conversion3/1 -> Demux1/1, Generate GPS Data/2("Vx, Vy, Vz")
  DCM/1 -> Data Type Conversion4/1
  Data Type Conversion4/1 -> Generate GPS Data/3(DCM)

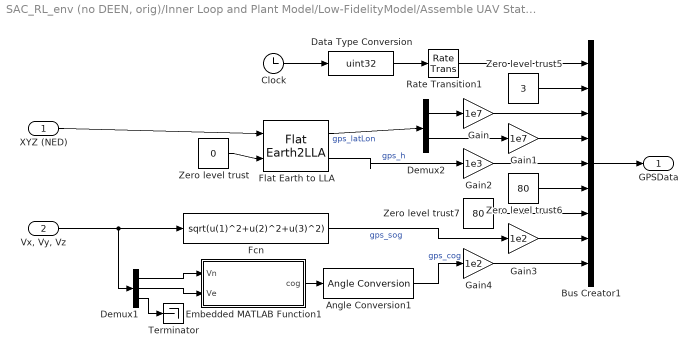
== system SAC_RL_env (no DEEN, orig)/Inner Loop and Plant Model/Low-FidelityModel/Assemble UAV State Bus/Generate GPS Data ==
  XYZ (NED) : Inport
  "Vx, Vy, Vz" : Inport  Port=2
  Angle Conversion1 : aerolibconvert2/Angle Conversion  IU=rad  OU=deg
  Bus Creator1 : BusCreator  Inputs=9  OutDataTypeStr=Bus: gps_raw_int  NonVirtualBus=on
      settings: InheritFromInputs=off
  Clock : Clock
      settings: AttributesFormatString=Decimation: %<Decimation>
  Data Type Conversion : DataTypeConversion  OutDataTypeStr=uint32  SaturateOnIntegerOverflow=off  RndMeth=Floor
  Demux1 : Demux  Outputs=3
  Demux2 : Demux  Outputs=2
  Embedded MATLAB Function1 : MATLAB Function  TreatAsAtomicUnit=on
  Fcn : Fcn  Expr=sqrt(u(1)^2+u(2)^2+u(3)^2)
  Flat Earth to LLA : FlatEarth2LLA  R=6378137  LL0=uavIC_latLon
  Gain : Gain  Gain=1e7  OutDataTypeStr=int32
  Gain1 : Gain  Gain=1e7  OutDataTypeStr=int32
  Gain2 : Gain  Gain=1e3  OutDataTypeStr=int32
  Gain3 : Gain  Gain=1e2  OutDataTypeStr=uint16
  Gain4 : Gain  Gain=1e2  OutDataTypeStr=uint16
  Rate Transition1 : RateTransition  OutPortSampleTime=0.005
  Terminator : Terminator
  Zero level trust : Constant  Value=0
      settings: AttributesFormatString=%<Value>
  Zero level trust5 : Constant  Value=3  OutDataTypeStr=uint8
      settings: AttributesFormatString=%<Value>
  Zero level trust6 : Constant  Value=80  OutDataTypeStr=uint16
      settings: AttributesFormatString=%<Value>
  Zero level trust7 : Constant  Value=80  OutDataTypeStr=uint16
      settings: AttributesFormatString=%<Value>
  GPSData : Outport  VectorParamsAs1DForOutWhenUnconnected=off
  wires:
  Demux1/3 -> Terminator/1
  Angle Conversion1/1 -> Gain4/1  "gps_cog"
  Embedded MATLAB Function1/1(cog) -> Angle Conversion1/1
  "Vx, Vy, Vz"/1 -> Demux1/1, Fcn/1
  Demux1/2 -> Embedded MATLAB Function1/2(Ve)
  Demux1/1 -> Embedded MATLAB Function1/1(Vn)
  Fcn/1 -> Gain3/1  "gps_sog"
  Flat Earth to LLA/1 -> Demux2/1  "gps_latLon"
  Zero level trust/1 -> Flat Earth to LLA/2
  XYZ (NED)/1 -> Flat Earth to LLA/1
  Clock/1 -> Data Type Conversion/1
  Flat Earth to LLA/2 -> Gain2/1  "gps_h"
  Demux2/1 -> Gain/1
  Demux2/2 -> Gain1/1
  Zero level trust5/1 -> Bus Creator1/2
  Gain1/1 -> Bus Creator1/4
  Zero level trust6/1 -> Bus Creator1/6
  Gain3/1 -> Bus Creator1/8
  Zero level trust7/1 -> Bus Creator1/7
  Gain4/1 -> Bus Creator1/9
  Gain2/1 -> Bus Creator1/5
  Gain/1 -> Bus Creator1/3
  Data Type Conversion/1 -> Rate Transition1/1
  Bus Creator1/1 -> GPSData/1
  Rate Transition1/1 -> Bus Creator1/1

== system SAC_RL_env (no DEEN, orig)/Inner Loop and Plant Model/Low-FidelityModel/Position and Acceleration Control/Attitude Control ==
  note: Use Heading Command to have
      | the copter turn into its heading.
      | Use Yaw Command to have the
      | copter turn towards the yaw given
      | by the Waypoint Mission
  Accel Cmd : Inport
  QuadRotorState : Inport  Port=2
  PositionCmd : Inport  Port=3
  Bus Creator : BusCreator  Inputs=4  OutDataTypeStr=Bus: uavGuidanceControlBus  NonVirtualBus=on
      settings: InheritFromInputs=off
  Bus Selector : BusSelector  OutputSignals=HeadingCmd,YawCmd
  Bus Selector1 : BusSelector  OutputSignals=EulerZYX
  Multirotor Acceleration Control : MATLAB Function  TreatAsAtomicUnit=on
  Multirotor Thrust Control : MATLAB Function  TreatAsAtomicUnit=on
  P Gain : Gain  Gain=1.1
  Selector1 : Selector  InputPortWidth=3  IndexOptions=Index vector (dialog)  Indices=[1]  OutputSizes=1
  Sum : Sum  Inputs=-+|
  Variant Source : VariantSource  VariantControls={useHeading ==1, useHeading ~= 1}
  dT Limit : Saturate  UpperLimit=1.2  LowerLimit=0
      settings: AttributesFormatString=[%<UpperLimit> %<LowerLimit>]
  phi Limit : Saturate  UpperLimit=25*pi/180  LowerLimit=-25*pi/180
      settings: AttributesFormatString=[%<UpperLimit> %<LowerLimit>]
  psi_dot Limit : Saturate  UpperLimit=30*pi/180  LowerLimit=-30*pi/180
      settings: AttributesFormatString=[%<UpperLimit> %<LowerLimit>]
  theta Limit : Saturate  UpperLimit=25*pi/180  LowerLimit=-25*pi/180
      settings: AttributesFormatString=[%<UpperLimit> %<LowerLimit>]
  Control Signal : Outport
  wires:
  Multirotor Thrust Control/1(thrust) -> dT Limit/1  "Thrust"
  QuadRotorState/1 -> Bus Selector1/1
  Multirotor Acceleration Control/1(roll) -> phi Limit/1  "Roll"
  Bus Creator/1 -> Control Signal/1
  dT Limit/1 -> Bus Creator/4  "thrust"
  P Gain/1 -> psi_dot Limit/1  "YawRate"
  Accel Cmd/1 -> Multirotor Thrust Control/1(acc), Multirotor Acceleration Control/1(acc)
  theta Limit/1 -> Bus Creator/2, Multirotor Thrust Control/2(pitch)  "Pitch"
  Sum/1 -> P Gain/1
  Selector1/1 -> Sum/1, Multirotor Acceleration Control/2(yaw)
  psi_dot Limit/1 -> Bus Creator/3  "YawRate"
  Bus Selector/2 -> Variant Source/2  "<YawCmd>"
  phi Limit/1 -> Bus Creator/1, Multirotor Thrust Control/3(roll)  "Roll"
  Variant Source/1 -> Sum/2
  Bus Selector1/1 -> Selector1/1  "<EulerZYX>"
  PositionCmd/1 -> Bus Selector/1
  Multirotor Acceleration Control/2(pitch) -> theta Limit/1  "Pitch"
  Bus Selector/1 -> Variant Source/1  "<HeadingCmd>"
